simulink model "Child_App"  (R2023a)
settings: Solver=FixedStepDiscrete  StartTime=0.0  StopTime=inf  RelTol=1e-3
libraries: androiduilib x5, androidsensorlib x3, androidaudiovideolib x2, androidcommunicationlib x2
settings Model: Creator=Aryan  LastModifiedBy=Aryan
settings OptimizationCC: EnhancedBackFolding=on  PassReuseOutputArgsAs=Individual arguments  ZeroExternalMemoryAtStartup=off  ZeroInternalMemoryAtStartup=off  MaxStackSize=64  OptimizeBlockOrder=speed  DifferentSizesBufferReuse=on  OptimizationCustomize=off  EfficientTunableParamExpr=on
settings DebuggingCC: ParameterTunabilityLossMsg=error
settings HardwareCC: ProdBitPerPointer=32  ProdBitPerSizeT=32  ProdBitPerPtrDiffT=32  ProdLargestAtomicInteger=Long  ProdLargestAtomicFloat=Double  ProdWordSize=32  ProdHWDeviceType=ARM Compatible->ARM Cortex
settings SFSimCC: MATLABDynamicMemAlloc=off
settings RTWCC: Description=Embedded Coder  SystemTargetFile=ert.tlc  HardwareBoard=Android Device  TLCOptions="-aInlineSetEventsForThisBaseRateFcn=TLC_FALSE -aSuppressMultiTaskScheduler=TLC_FALSE  -aRateBasedStepFcn=0"  TemplateMakefile=ert_default_tmf  RTWVerbose=off  Toolchain=Android SDK/NDK Tools  BuildConfiguration=Faster Runs
settings CodeAppCC: ForceParamTrailComments=on  IgnoreCustomStorageClasses=off  OperatorAnnotations=on  SimulinkDataObjDesc=on  SFDataObjDesc=on  InsertBlockDesc=on

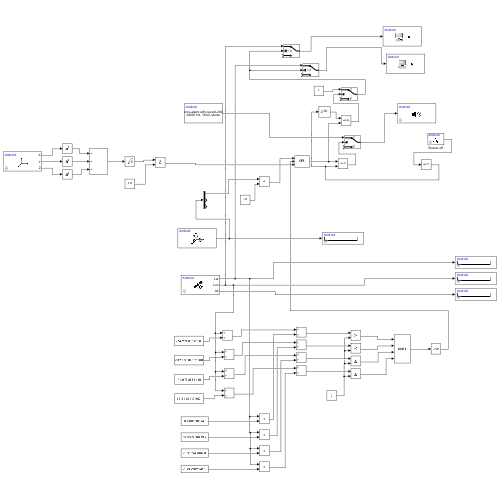
[thumbnail: Simulink's stored preview of the top-level diagram]
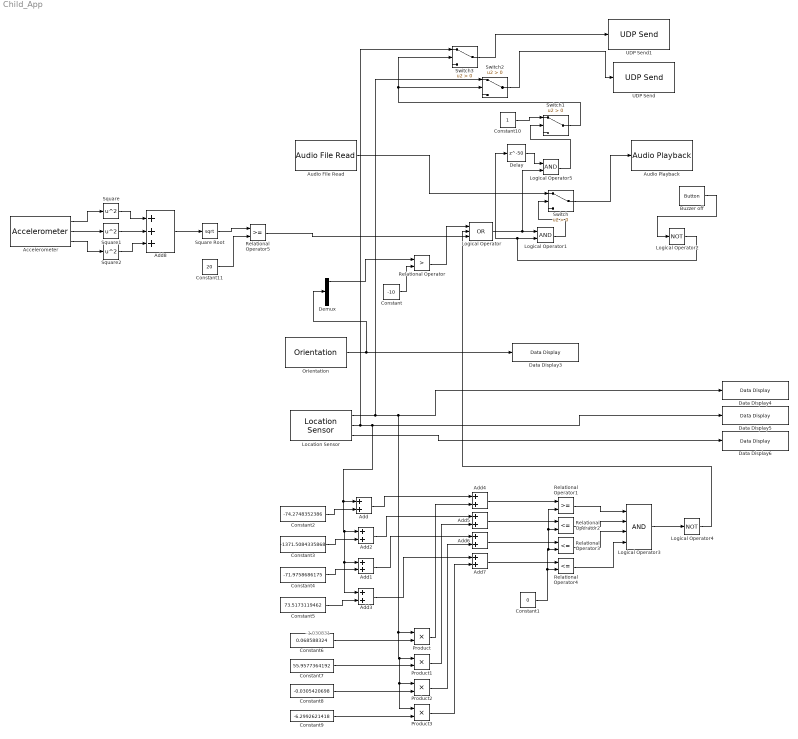
== system Child_App ==
  note: -1.030831
  Accelerometer : androidsensorlib/Accelerometer  OutputVector=off  SampleTime=0.1  BlockPlatform=Android
  Add{,1..7} (8 alike) : Sum
  Add8 : Sum  Inputs=+++
  Audio File Read : androidaudiovideolib/Audio File Read  FileName=C:\Users\aryan\Downloads\emergency-alarm-with-reverb-29431.wav  FrameSize=2400
  Audio Playback : androidaudiovideolib/Audio Playback  SampleFreq=24000  AudioSamplingFreq=24000  SampleTime=0.1  DeviceStr=0  QueueDuration=0  BlockPlatform=Android
  Buzzer off : androiduilib/Button  ButtonState=Not pressed  ButtonId=Child_App/Buzzer_off  State=off  SampleTime=0.1  BlockPlatform=Android
  Constant : Constant  Value=-10
  Constant1 : Constant  Value=0
  Constant10 : Constant
  Constant11 : Constant  Value=20
  Constant2 : Constant  Value=-74.2748352386
  Constant3 : Constant  Value=-1371.5084335868
  Constant4 : Constant  Value=-71.9758686175
  Constant5 : Constant  Value=73.5173119462
  Constant6 : Constant  Value=0.068588324
  Constant7 : Constant  Value=55.9577364192
  Constant8 : Constant  Value=-0.0305420698
  Constant9 : Constant  Value=-6.2992621418
  Data Display3 : androiduilib/Data Display  DataDisplayId=Child_App/Data_Display3  Format=Float  Precision=6  SimulateUsing=Code generation  blockPlatform=Android
  Data Display4 : androiduilib/Data Display  DataDisplayId=Child_App/Data_Display4  Format=Float  Precision=6  SimulateUsing=Code generation  blockPlatform=Android
  Data Display5 : androiduilib/Data Display  DataDisplayId=Child_App/Data_Display5  Format=Float  Precision=6  SimulateUsing=Code generation  blockPlatform=Android
  Data Display6 : androiduilib/Data Display  DataDisplayId=Child_App/Data_Display6  Format=Float  Precision=6  SimulateUsing=Code generation  blockPlatform=Android
  Delay : Delay  DelayLength=50  InitialCondition=0
  Demux : Demux  Outputs=3
  Location Sensor : androidsensorlib/Location Sensor  OutputVector=off  SampleTime=0.1  BlockPlatform=Android
  Logical Operator : Logic  Operator=OR  Inputs=3  AllPortsSameDT=off  OutDataTypeStr=boolean
  Logical Operator1 : Logic  AllPortsSameDT=off  OutDataTypeStr=boolean
  Logical Operator2 : Logic  Operator=NOT  AllPortsSameDT=off  OutDataTypeStr=boolean
  Logical Operator3 : Logic  Inputs=4  AllPortsSameDT=off  OutDataTypeStr=boolean
  Logical Operator4 : Logic  Operator=NOT  AllPortsSameDT=off  OutDataTypeStr=boolean
  Logical Operator5 : Logic  AllPortsSameDT=off  OutDataTypeStr=boolean
  Orientation : androidsensorlib/Orientation  SampleTime=0.1
  Product{,1..3} (4 alike) : Product
  Relational Operator : RelationalOperator  Operator=>  OutDataTypeStr=boolean  RndMeth=Simplest  InputSameDT=off
  Relational Operator1 : RelationalOperator  OutDataTypeStr=boolean  RndMeth=Simplest  InputSameDT=off
  Relational Operator2 : RelationalOperator  Operator=<=  OutDataTypeStr=boolean  RndMeth=Simplest  InputSameDT=off
  Relational Operator3 : RelationalOperator  Operator=<=  OutDataTypeStr=boolean  RndMeth=Simplest  InputSameDT=off
  Relational Operator4 : RelationalOperator  Operator=<=  OutDataTypeStr=boolean  RndMeth=Simplest  InputSameDT=off
  Relational Operator5 : RelationalOperator  OutDataTypeStr=boolean  RndMeth=Simplest  InputSameDT=off
  Square : Math  Operator=square
  Square Root : Sqrt
  Square1 : Math  Operator=square
  Square2 : Math  Operator=square
  Switch{,1..3} (4 alike) : Switch  Criteria=u2 > Threshold  SaturateOnIntegerOverflow=off  InputSameDT=off
  UDP Send : androidcommunicationlib/UDP Send  remoteURL='10.7.0.77'  remotePort=25000  localURL='0.0.0.0'  localPortSource=Automatically determine  localPort=-1  sampletime=-1  blockPlatform=Android  separateLengthPort=0
  UDP Send1 : androidcommunicationlib/UDP Send  remoteURL='10.7.0.77'  remotePort=25001  localURL='0.0.0.0'  localPortSource=Automatically determine  localPort=-1  sampletime=-1  blockPlatform=Android  separateLengthPort=0
  wires:
  Relational Operator/1 -> Logical Operator/1
  Location Sensor/1 -> Switch2/1, Product3/1, Product2/1, Product1/1, Product/1, Data Display4/1
  Location Sensor/2 -> Switch3/1, Add3/1, Add1/1, Add2/1, Add/1, Data Display5/1
  Location Sensor/3 -> Data Display6/1
  Switch/1 -> Audio Playback/1
  Audio File Read/1 -> Switch/1
  Constant/1 -> Relational Operator/2
  Orientation/1 -> Data Display3/1, Demux/1
  Demux/1 -> Relational Operator/1
  Logical Operator/1 -> Logical Operator5/2, Logical Operator1/1
  Logical Operator1/1 -> Switch/2
  Logical Operator2/1 -> Delay/1, Logical Operator1/2
  Buzzer off/1 -> Logical Operator2/1
  Logical Operator3/1 -> Logical Operator4/1
  Logical Operator4/1 -> Logical Operator/2
  Constant1/1 -> Relational Operator1/2, Relational Operator2/2, Relational Operator3/2, Relational Operator4/2
  Relational Operator1/1 -> Logical Operator3/1
  Relational Operator2/1 -> Logical Operator3/2
  Relational Operator3/1 -> Logical Operator3/3
  Relational Operator4/1 -> Logical Operator3/4
  Constant5/1 -> Add3/2
  Constant4/1 -> Add1/2
  Constant3/1 -> Add2/2
  Constant2/1 -> Add/2
  Constant6/1 -> Product/2
  Constant7/1 -> Product1/2
  Constant8/1 -> Product2/2
  Constant9/1 -> Product3/2
  Add4/1 -> Relational Operator1/1
  Add7/1 -> Relational Operator4/1
  Add6/1 -> Relational Operator3/1
  Add5/1 -> Relational Operator2/1
  Product/1 -> Add4/2
  Product1/1 -> Add5/2
  Product2/1 -> Add6/2
  Product3/1 -> Add7/2
  Add/1 -> Add4/1
  Add2/1 -> Add5/1
  Add1/1 -> Add6/1
  Add3/1 -> Add7/1
  Constant10/1 -> Switch1/1
  Delay/1 -> Logical Operator5/1
  Logical Operator5/1 -> Switch1/2
  Switch1/1 -> Switch3/2, Switch2/2
  Switch2/1 -> UDP Send/1
  Switch3/1 -> UDP Send1/1
  Accelerometer/1 -> Square/1
  Accelerometer/2 -> Square1/1
  Accelerometer/3 -> Square2/1
  Square/1 -> Add8/1
  Square1/1 -> Add8/2
  Square2/1 -> Add8/3
  Add8/1 -> Square Root/1
  Square Root/1 -> Relational Operator5/1
  Constant11/1 -> Relational Operator5/2
  Relational Operator5/1 -> Logical Operator/3
